simulink model "planar_2dof_ik"  (R2025a)
settings: Solver=VariableStepAuto  StartTime=0.0  StopTime=10.0  RelTol=1e-3
settings Model: Creator=hocke  LastModifiedBy=hocke

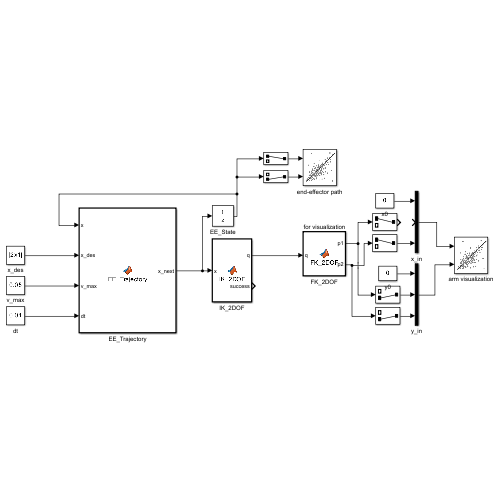
[thumbnail: Simulink's stored preview of the top-level diagram]
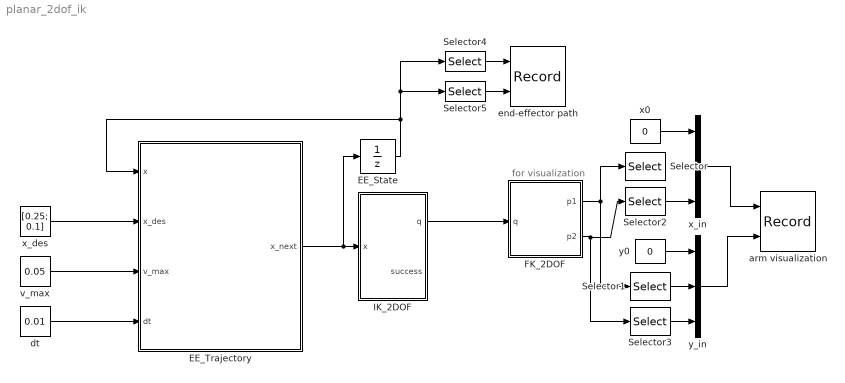
== system planar_2dof_ik ==
  note: for visualization
  EE_State : UnitDelay  InitialCondition=[0.2; 0]  SampleTime=-1  HasFrameUpgradeWarning=on
  "EE_Trajectory " : MATLAB Function  TreatAsAtomicUnit=on
  FK_2DOF : MATLAB Function  TreatAsAtomicUnit=on
  "IK_2DOF " : MATLAB Function  TreatAsAtomicUnit=on
  Selector : Selector  InputPortWidth=2  IndexOptions=Index vector (dialog)  Indices=1  OutputSizes=1
  Selector1 : Selector  InputPortWidth=2  IndexOptions=Index vector (dialog)  Indices=2  OutputSizes=1
  Selector2 : Selector  InputPortWidth=2  IndexOptions=Index vector (dialog)  Indices=1  OutputSizes=1
  Selector3 : Selector  InputPortWidth=2  IndexOptions=Index vector (dialog)  Indices=2  OutputSizes=1
  Selector4 : Selector  InputPortWidth=2  IndexOptions=Index vector (dialog)  Indices=1  OutputSizes=1
  Selector5 : Selector  InputPortWidth=2  IndexOptions=Index vector (dialog)  Indices=2  OutputSizes=1
  arm visualization : Record  NumPorts=2.0  FileSettingsInternal="{\"entries\":[{\"content\":{\"excelSettings\":{\"content\":{},\"type\":\"Streamout.ExcelSettings\"},\"parquetSettings\":{\"content\":{},\"type\":\"Streamout.ParquetSettings\"}},\"type\":\"Streamout.FileSettingStorage\",\"uuid\":\"\"}],\"packageUris\":[\"http:\\/\\/schema.mathworks.com\\/mf0\\/streamout_blocks\\/R2020a\"],\"version\":\"1.0\"}"  FrameSettings=[0, 0]  Layout=[1 1]  SignalsInternal="{\"entries\":[{\"content\":{\"signals\":[{\"content\":{\"blockPath\":[],\"dimensions\":[3],\"domain\":\"\",\"hasChildren\":true,\"lineColor\":\"#0072bd\",\"lineWidth\":2,\"port\":1,\"sid\":[\"\"],\"signalID\":1,\"signalName\":\"x_in\"},\"type\":\"RecordBlkView.Signal\",\"uuid\":\"\"},{\"content\":{\"blockPath\":[],\"channel\":[1],\"dimensions\":[3],\"domain\":\"\",\"lineColor\":\"#b746ff\",\"lineWidth\":2,\"parentID\":1,\"plots\":[ 1 ],\"port\":1,\"sid\":[\"\"],\"signalID\":2,\"signalName\":\"x_in\"},\"type\":\"RecordBlkView.Signal\",\"uuid\":\"\"},{\"content\":{\"blockPath\":[],\"dimensions\":[3],\"domain\":\"\",\"hasChildren\":true,\"lineColor\":\"#edb120\",\"lineWidth\":2,\"port\":2,\"sid\":[\"\"],\"signalID\":3,\"signalName\":\"y_in\"},\"type\":\"RecordBlkView.Signal\",\"uuid\":\"\"},{\"content\":{\"blockPath\":[],\"channel\":[1],\"dimensions\":[3],\"domain\":\"\",\"lineColor\":\"#ff13a6\",\"lineWidth\":2,\"parentID\":3,\"plots\":[ 1 ],\"port\":2,\"sid\":[\"\"],\"signalID\":4,\"signalName\":\"y_in\"},\"type\":\"RecordBlkView.Signal\",\"uuid\":\"\"},{\"content\":{\"blockPath\":[],\"channel\":[2],\"dimensions\":[3],\"domain\":\"\",\"lineColor\":\"#0072bd\",\"lineWidth\":2,\"parentID\":1,\"plots\":[ 1 ],\"port\":1,\"sid\":[\"\"],\"signalID\":5,\"signalName\":\"x_in\"},\"type\":\"RecordBlkView.Signal\",\"uuid\":\"\"},{\"content\":{\"blockPath\":[],\"channel\":[3],\"dimensions\":[3],\"domain\":\"\",\"lineColor\":\"#d95319\",\"lineWidth\":2,\"parentID\":1,\"plots\":[ 1 ],\"port\":1,\"sid\":[\"\"],\"signalID\":6,\"signalName\":\"x_in\"},\"type\":\"RecordBlkView.Signal\",\"uuid\":\"\"},{\"content\":{\"blockPath\":[],\"channel\":[2],\"dimensions\":[3],\"domain\":\"\",\"lineColor\":\"#edb120\",\"lineWidth\":2,\"parentID\":3,\"plots\":[ 1 ],\"port\":2,\"sid\":[\"\"],\"signalID\":7,\"signalName\":\"y_in\"},\"type\":\"RecordBlkView.Signal\",\"uuid\":\"\"},{\"content\":{\"blockPath\":[],\"channel\":[3],\"dimensions\":[3],\"domain\":\"\",\"lineColor\":\"#7e2f8e\",\"lineWidth\":2,\"parentID\":3,\"plots\":[ 1 ],\"port\":2,\"sid\":[\"\"],\"signalID\":8,\"signalName\":\"y_in\"},\"type\":\"RecordBlkView.Signal\",\"uuid\":\"\"}]},\"type\":\"RecordBlkView.InputSignals\",\"uuid\":\"\"}],\"packageUris\":[\"http:\\/\\/schema.mathworks.com\\/mf0\\/streamout_blocks\\/R2020a\"],\"version\":\"1.0\"}"  VisualizationBindings="{\"xyplotplugin\":{\"info\":[{\"series\":[{\"bindingParametersList\":[{\"parameter\":\"X-Axis\",\"signalID\":2,\"signalName\":\"x_in(1)\"},{\"parameter\":\"Y-Axis\",\"signalID\":4,\"signalName\":\"y_in(1)\"}],\"seriesID\":0},{\"bindingParametersList\":[{\"parameter\":\"X-Axis\",\"signalID\":5,\"signalName\":\"x_in(2)\"},{\"parameter\":\"Y-Axis\",\"signalID\":7,\"signalName\":\"y_in(2)\"}],\"seriesID\":1},{\"bindingParametersList\":[{\"parameter\":\"X-Axis\",\"signalID\":6,\"signalName\":\"x_in(3)\"},{\"parameter\":\"Y-Axis\",\"signalID\":8,\"signalName\":\"y_in(3)\"}],\"seriesID\":2}],\"subplotID\":1}]}}"  CompatibilityTag=XY
  dt : Constant  Value=0.01
  end-effector path : Record  NumPorts=2.0  FileSettingsInternal="{\"entries\":[{\"content\":{\"excelSettings\":{\"content\":{},\"type\":\"Streamout.ExcelSettings\"},\"parquetSettings\":{\"content\":{},\"type\":\"Streamout.ParquetSettings\"}},\"type\":\"Streamout.FileSettingStorage\",\"uuid\":\"\"}],\"packageUris\":[\"http:\\/\\/schema.mathworks.com\\/mf0\\/streamout_blocks\\/R2020a\"],\"version\":\"1.0\"}"  FrameSettings=[0, 0]  Layout=[1 1]  SignalsInternal="{\"entries\":[{\"content\":{\"signals\":[{\"content\":{\"blockPath\":[],\"dimensions\":[1,1],\"domain\":\"\",\"lineColor\":\"#a2142f\",\"plots\":[ 1 ],\"port\":1,\"sid\":[\"\"],\"signalID\":1,\"signalName\":\"Selector4\"},\"type\":\"RecordBlkView.Signal\",\"uuid\":\"\"},{\"content\":{\"blockPath\":[],\"dimensions\":[1,1],\"domain\":\"\",\"lineColor\":\"#139fff\",\"plots\":[ 1 ],\"port\":2,\"sid\":[\"\"],\"signalID\":2,\"signalName\":\"Selector5\"},\"type\":\"RecordBlkView.Signal\",\"uuid\":\"\"}]},\"type\":\"RecordBlkView.InputSignals\",\"uuid\":\"\"}],\"packageUris\":[\"http:\\/\\/schema.mathworks.com\\/mf0\\/streamout_blocks\\/R2020a\"],\"version\":\"1.0\"}"  VisualizationBindings="{\"xyplotplugin\":{\"info\":[{\"series\":[{\"bindingParametersList\":[{\"parameter\":\"X-Axis\",\"signalID\":1,\"signalName\":\"Selector4\"},{\"parameter\":\"Y-Axis\",\"signalID\":2,\"signalName\":\"Selector5\"},{\"parameter\":\"X-Axis\",\"signalID\":1,\"signalName\":\"Selector4\"},{\"parameter\":\"Y-Axis\",\"signalID\":2,\"signalName\":\"Selector5\"}],\"seriesID\":0}],\"subplotID\":1}]}}"  CompatibilityTag=XY
  v_max : Constant  Value=0.05
  x0 : Constant  Value=0
  x_des : Constant  Value=[0.25; 0.1]
  x_in : Mux  Inputs=3
  y0 : Constant  Value=0
  y_in : Mux  Inputs=3
  wires:
  x_des/1 -> "EE_Trajectory "/2(x_des)
  v_max/1 -> "EE_Trajectory "/3(v_max)
  dt/1 -> "EE_Trajectory "/4(dt)
  EE_State/1 -> Selector5/1, Selector4/1, "EE_Trajectory "/1(x)
  "EE_Trajectory "/1(x_next) -> "IK_2DOF "/1(x), EE_State/1
  "IK_2DOF "/1(q) -> FK_2DOF/1(q)
  x0/1 -> x_in/1
  x_in/1 -> arm visualization/1
  y_in/1 -> arm visualization/2
  y0/1 -> y_in/1
  Selector4/1 -> end-effector path/1
  Selector5/1 -> end-effector path/2
  FK_2DOF/1(p1) -> Selector/1, Selector1/1
  Selector1/1 -> y_in/2
  FK_2DOF/2(p2) -> Selector2/1, Selector3/1
  Selector3/1 -> y_in/3
  Selector2/1 -> x_in/3

== matlab function planar_2dof_ik/IK_2DOF  ==
  data: x input; q output; success output
function [q, success] = IK_2DOF(x)
%#codegen

L1 = 0.2;
L2 = 0.2;

X = x(1);
Y = x(2);

r2 = X^2 + Y^2;
c2 = (r2 - L1^2 - L2^2)/(2*L1*L2);

if abs(c2) > 1
    q = [0;0];
    success = false;
    return;
end

s2 = sqrt(1 - c2^2);
q2 = atan2(s2, c2);

k1 = L1 + L2*c2;
k2 = L2*s2;
q1 = atan2(Y, X) - atan2(k2, k1);

q = [q1; q2];
success = true;
end

== matlab function planar_2dof_ik/EE_Trajectory  ==
  data: x input; x_next output; x_des input; v_max input; dt input
function x_next = EE_Trajectory(x, x_des, v_max, dt)
%#codegen

dx = x_des - x;
dist = norm(dx);

if dist < 1e-6
    x_next = x;
    return;
end

step = min(dist, v_max*dt);
x_next = x + step * dx / dist;
end

== matlab function planar_2dof_ik/FK_2DOF ==
  data: q input; p1 output; p2 output
function [p1, p2] = FK_2DOF(q)
L1 = 0.2;
L2 = 0.2;

q1 = q(1);
q2 = q(2);

p1 = [L1*cos(q1); L1*sin(q1)];
p2 = p1 + [L2*cos(q1+q2); L2*sin(q1+q2)];
end
